simulink model "model_virtualpartner_bros"  (R2016b)
settings: Solver=FixedStepDiscrete  StartTime=0.0  StopTime=inf  FixedStep=sampleTime  RelTol=1e-3
PostLoadFcn:
  | % load model parameters
  | % pname = fileparts(get_param('model_base_bros','filename'));
  | % run([pname  '\parameters_base_model_bros.m']);
  | parameters_virtualpartner_bros;
  | 
  | % set requested state
  | set_param('model_virtualpartner_bros/Requested state','Value',num2str(0));
InitFcn:
  | % load model parameters
  | % pname = fileparts(get_param('model_base_bros','filename'));
  | % run([pname  '\parameters_base_model_bros.m']);
  | parameters_virtualpartner_bros;
  | 
  | % set requested state
  | set_param('model_virtualpartner_bros/Requested state','Value',num2str(0));
StartFcn:
  | % load model parameters
  | % pname = fileparts(get_param('model_base_bros','filename'));
  | % run([pname  '\parameters_base_model_bros.m']);
  | parameters_virtualpartner_bros;
  | 
  | % set requested state
  | set_param('model_virtualpartner_bros/Requested state','Value',num2str(0));
StopFcn:
  | % switch off data logger (to hopefully avoid corrupt files). TwinCAT doesn't properly switch off the logger when shutting down the model
  | % no idea if this'll work.
  | set_param('model_virtualpartner_bros/Record data (1 = yes, 0 = no)','Value',num2str(0));
values from neighbouring files (symbols this model uses):
  Ax = [0.0286583637244 0.0270981680387 0.0234505258969 0.0179991434705]    [data_target_signal.mat]    (also in data_target_signal3.mat = [0.0333782282668 0.0245436264839 0.0161138842629 0.007570500; data_target_signal4.mat = [0.0269405878553 0.022932388404 0.0177213023263 0.0101459636; data_target_signal5.mat = [0.0280601816416 0.0238854099083 0.0184577621273 0.010567608)
  Ay = [0.0270981680387 0.0253254894496 0.0215637914741 0.0163904070646]    [data_target_signal.mat]    (also in data_target_signal3.mat = [0.0316365733513 0.022903298684 0.0150378639378 0.0071644979; data_target_signal4.mat = [0.0262391735578 0.0220449066546 0.0169202788634 0.009702651; data_target_signal5.mat = [0.0273296180511 0.0229610462966 0.0176234498254 0.010105872)
  FFMatrix = [0 -20; 20 0]*-1    [parameters_base_model_bros.m]    (also in parameters_model_virtualpartner_bros.m = -[0 -15; 15 0]; parameters_virtualpartner_bros.m = -[0 -15; 15 0])
  Lb = 0.07    [parameters_base_model_bros.m]    (also in parameters_model_virtualpartner_bros.m; parameters_virtualpartner_bros.m)
  Lf = 0.238    [parameters_base_model_bros.m]    (also in parameters_model_virtualpartner_bros.m; parameters_virtualpartner_bros.m)
  Lu = 0.153    [parameters_base_model_bros.m]    (also in parameters_model_virtualpartner_bros.m; parameters_virtualpartner_bros.m)
  nx = [3 4 6 9]    [data_target_signal.mat]    (also in data_target_signal3.mat = [6 11 17 29]; data_target_signal4.mat = [6 11 17 29]; data_target_signal5.mat = [6 11 17 29])
  ny = [4 5 7 10]    [data_target_signal.mat]    (also in data_target_signal3.mat = [7 12 18 30]; data_target_signal4.mat = [7 12 18 30]; data_target_signal5.mat = [7 12 18 30])
  phx = [-7.77441521106 -8.5348832042 -4.36104325862 -3.78796037329]    [data_target_signal.mat]    (also in data_target_signal3.mat = [3.56575266464 -2.00335535647 1.65538939475 0.759048650391]; data_target_signal4.mat = [-7.8125213649 -4.12353525545 6.3256632478 -1.21163926456]; data_target_signal5.mat = [2.80153374524 -3.20046313064 -3.48286348128 -10.5236026319])
  phy = [-0.714244784373 -3.45250659197 3.9180169666 4.93073057512]    [data_target_signal.mat]    (also in data_target_signal3.mat = [9.98760310067 -6.16453798136 -6.84315611985 5.69872885715]; data_target_signal4.mat = [6.54917483844 9.11210927212 4.8993819932 2.56946947623]; data_target_signal5.mat = [-1.40862004251 -1.67034924642 8.20266618674 -4.37156725072])
  sampleTime = 0.001    [parameters_base_model_bros.m]    (also in parameters_model_virtualpartner_bros.m; parameters_virtualpartner_bros.m)
undefined symbols (not defined in the file or in its folder): BROS1, BROS2, VP
libraries: simulink x29, LibraryFM x14, VariousBlocksLibrary x7, simulink_extras x1
(part 3 of 3)

== system model_virtualpartner_bros/Robot2/DataToEtherCAT/WorkspacePositionGuard ==
  note: Check internal angles
  note: Check whether endpoint position is within the predefined workspace
      | (ellipse)
  note: Check for singularity of joint configuration by checking
      | the condition number. When it exceeds a certain value, go to a safe mode
      | For now, this means disabling the actuators.
      | Note that the boundaries set using admittance should prohibit this from happening.
      | However, if sometjhing really goes wrong, this is a safe guard
  BusRobot : Inport
  StateSystem : Inport  Port=2
  AvoidAlgebraicLoop : Memory
  Bus Selector : BusSelector  OutputSignals=xOpSpace.x,xOpSpace.conditioning,qJointSpace.q_all
  CheckInternalAngles : MATLAB Function  TreatAsAtomicUnit=on
  Compare To Constant : simulink/Logic and Bit Operations/Compare To Constant  relop=>  const=4  OutDataTypeStr=boolean
  Compare To Constant1 : simulink/Logic and Bit Operations/Compare To Constant  relop=>=  const=2.75  OutDataTypeStr=boolean
  Data Type Conversion1 : DataTypeConversion  OutDataTypeStr=boolean
  Data Type Conversion2 : DataTypeConversion  Commented=through  OutDataTypeStr=int32
  Data Type Conversion4 : DataTypeConversion  OutDataTypeStr=boolean
  Detect Change : simulink/Logic and Bit Operations/Detect Change  vinit=0  InputProcessing=Inherited  OutDataTypeStr=boolean
  EndpointPositionGuard : MATLAB Function  TreatAsAtomicUnit=on
  LatchRising : LibraryFM/Utilities/LatchRising  ic=0
  Logical Operator : Logic  Operator=OR  AllPortsSameDT=off  OutDataTypeStr=boolean
  Mux : Mux  Inputs=2
  ShowWorkspaceErrorLatched : Display
  WorkspaceLastError : Display
  WorkspaceError : Outport
  WorkspaceErrorLatched : Outport  Port=2
  wires:
  BusRobot/1 -> Bus Selector/1
  Bus Selector/1 -> EndpointPositionGuard/2(xe)  "<x>"
  LatchRising/1 -> Data Type Conversion2/1
  EndpointPositionGuard/1(error) -> Data Type Conversion1/1
  Mux/1 -> AvoidAlgebraicLoop/1, WorkspaceLastError/1
  Detect Change/1 -> LatchRising/Trigger
  AvoidAlgebraicLoop/1 -> WorkspaceError/1, Detect Change/1, LatchRising/1
  Compare To Constant/1 -> EndpointPositionGuard/1(correctState)
  Bus Selector/2 -> Compare To Constant1/1  "<conditioning>"
  StateSystem/1 -> Compare To Constant/1
  Data Type Conversion2/1 -> WorkspaceErrorLatched/1, ShowWorkspaceErrorLatched/1
  CheckInternalAngles/1(angleError) -> Data Type Conversion4/1
  Bus Selector/3 -> CheckInternalAngles/1(theta)  "<q_all>"
  Data Type Conversion4/1 -> Mux/2
  Logical Operator/1 -> Mux/1
  Data Type Conversion1/1 -> Logical Operator/1
  Compare To Constant1/1 -> Logical Operator/2

== system model_virtualpartner_bros/Experiment & Haptics/Admittance // Virtual model1/Virtual Model/HoldFirstSampleOnEnable ==
  note: These blocks hold the first sample of the input
      | when the block is enabled (through the action port)
  x : Inport
  Enable : EnablePort  StatesWhenEnabling=reset
  Counter Free-Running : simulink/Sources/Counter Free-Running  NumBits=32  tsamp=-1
  Display : Display
  Memory1 : Memory
  Switch : Switch  Threshold=1
  x0 : Outport
  wires:
  Switch/1 -> Display/1, Memory1/1, x0/1
  Memory1/1 -> Switch/1
  Counter Free-Running/1 -> Switch/2
  x/1 -> Switch/3

== system model_virtualpartner_bros/Experiment & Haptics/Admittance // Virtual model1/Virtual Model/HoldFirstSampleOnEnable1 ==
  note: These blocks hold the first sample of the input
      | when the block is enabled (through the action port)
  x : Inport
  Enable : EnablePort  StatesWhenEnabling=reset
  Counter Free-Running : simulink/Sources/Counter Free-Running  NumBits=32  tsamp=-1
  Display : Display
  Memory1 : Memory
  Switch : Switch  Threshold=1
  x0 : Outport
  wires:
  Switch/1 -> Display/1, Memory1/1, x0/1
  Memory1/1 -> Switch/1
  Counter Free-Running/1 -> Switch/2
  x/1 -> Switch/3

== system model_virtualpartner_bros/Experiment & Haptics/Admittance // Virtual model1/Virtual Model/simple Virtual partner LQG2 ==
  target : Inport
  L_VP : Inport  Port=2
  ExecuteVP : Inport  Port=3
  Fs : Inport  Port=4
  CoAimmstant : Constant  Value=VP.Aim
  CoAimmstant1 : Constant  Value=VP.B
  CoAimmstant2 : Constant  Value=VP.Ae
  CoAimmstant3 : Constant  Value=VP.H
  CoAimmstant5 : Constant  Value=VP.Ov
  CoAimmstant6 : Constant  Value=VP.Ow
  CoAimmstant8 : Constant  Value=VP.Ndelay
  Compare To Zero : simulink/Logic and Bit Operations/Compare To Zero  relop=>  OutDataTypeStr=boolean
  Constant : Constant  Value=VP.m
  Data Type Conversion : DataTypeConversion  OutDataTypeStr=double
  Mux : Mux  Inputs=2
  Product : Product
  Virtual Partner LQG : MATLAB Function  TreatAsAtomicUnit=on
  select [px vx py vy] from state vector : Selector  InputPortWidth=14  IndexOptions=Index vector (dialog)  Indices=[1 2 3 4]  OutputSizes=1
  xVP_prev1 : UnitDelay  InitialCondition=VP.x0  SampleTime=-1
  xhatp1 : Delay  DelayLength=1
  y1 : Delay  DelayLength=100
  x_VP : Outport
  data : Outport  Port=2
  wires:
  CoAimmstant5/1 -> Virtual Partner LQG/5(Ov)
  CoAimmstant2/1 -> Virtual Partner LQG/1(Ae)
  CoAimmstant3/1 -> Virtual Partner LQG/4(H)
  CoAimmstant1/1 -> Virtual Partner LQG/3(B)
  L_VP/1 -> Virtual Partner LQG/9(L)
  CoAimmstant/1 -> Virtual Partner LQG/2(Aim)
  xVP_prev1/1 -> Virtual Partner LQG/11(xVP_prev)
  CoAimmstant6/1 -> Virtual Partner LQG/6(Ow)
  Virtual Partner LQG/2(y) -> Mux/1, y1/1
  y1/1 -> Virtual Partner LQG/12(y_delay)
  Virtual Partner LQG/3(xhatp) -> Mux/2, xhatp1/1
  xhatp1/1 -> Virtual Partner LQG/13(xhatp_delay)
  CoAimmstant8/1 -> Virtual Partner LQG/7(Ndelay)
  target/1 -> Virtual Partner LQG/8(target)
  Virtual Partner LQG/1(x_VP) -> xVP_prev1/1, select [px vx py vy] from state vector/1
  ExecuteVP/1 -> Compare To Zero/1
  Compare To Zero/1 -> Data Type Conversion/1
  Product/1 -> x_VP/1
  select [px vx py vy] from state vector/1 -> Product/1
  Data Type Conversion/1 -> Product/2
  Mux/1 -> data/1
  Fs/1 -> Virtual Partner LQG/10(Fs)
  Constant/1 -> Virtual Partner LQG/14(m_vp)

== system model_virtualpartner_bros/Experiment & Haptics/Admittance // Virtual model1/Virtual partner control law/Triggered Subsystem ==
  VPModelParams : Inport
  Trigger : TriggerPort  VariantControl=Variant
  CoAimmstant : Constant  Value=VP.Aim
  CoAimmstant1 : Constant  Value=VP.B
  MATLAB Function : MATLAB Function  TreatAsAtomicUnit=on
  FBGains : Outport  InitialOutput=zeros(2,14)
  wires:
  VPModelParams/1 -> MATLAB Function/1(modelparams)
  MATLAB Function/1(L) -> FBGains/1
  CoAimmstant/1 -> MATLAB Function/2(Aim_vp)
  CoAimmstant1/1 -> MATLAB Function/3(B_vp)

== system model_virtualpartner_bros/Experiment & Haptics/Admittance // Virtual model1/Virtual partner control law/Triggered Subsystem1 ==
  VPModelParams : Inport
  Trigger : TriggerPort  VariantControl=Variant
  CoAimmstant : Constant  Value=VP.Aim
  CoAimmstant1 : Constant  Value=VP.B
  MATLAB Function : MATLAB Function  TreatAsAtomicUnit=on
  FBGains : Outport  InitialOutput=zeros(2,14)
  wires:
  VPModelParams/1 -> MATLAB Function/1(modelparams)
  MATLAB Function/1(L) -> FBGains/1
  CoAimmstant/1 -> MATLAB Function/2(Aim_vp)
  CoAimmstant1/1 -> MATLAB Function/3(B_vp)

== system model_virtualpartner_bros/Robot1/Controller_PD/at home/HoldFirstSampleOnEnable ==
  note: These blocks hold the first sample of the input
      | when the block is enabled (through the action port)
  x : Inport
  Enable : EnablePort  StatesWhenEnabling=reset
  Counter Free-Running : simulink/Sources/Counter Free-Running  NumBits=32  tsamp=-1
  Memory1 : Memory
  Signal Conversion : SignalConversion  OverrideOpt=off
  Switch : Switch  Threshold=1
  x0 : Outport
  wires:
  x/1 -> Switch/3
  Counter Free-Running/1 -> Switch/2
  Memory1/1 -> Switch/1
  Switch/1 -> Signal Conversion/1, Memory1/1
  Signal Conversion/1 -> x0/1

== system model_virtualpartner_bros/Robot1/DataFromEtherCAT/Calculate Arrange Joint and Op Space/forward kinematics ==
  JointPosition_rad : Inport  PortDimensions=[2 1]
  JointVelocity_rads : Inport  Port=2  PortDimensions=[2 1]
  JointAcceleration_rads2 : Inport  Port=3  PortDimensions=[2 1]
  Je : MATLAB Function  TreatAsAtomicUnit=on
  Jedot : MATLAB Function  TreatAsAtomicUnit=on
  Product : Product  Multiplication=Matrix(*)
  calculate xddot : MATLAB Function  TreatAsAtomicUnit=on
  forward kinematics : MATLAB Function  TreatAsAtomicUnit=on
  x : Outport
  xdot : Outport  Port=2
  xddot : Outport  Port=3
  J : Outport  Port=4
  Jdot : Outport  Port=5
  wires:
  JointPosition_rad/1 -> forward kinematics/1(q), Jedot/1(q), Je/1(q)
  Je/1(Je) -> calculate xddot/3(J), Product/1, J/1
  JointVelocity_rads/1 -> calculate xddot/2(qdot), Product/2, Jedot/2(qdot)
  Jedot/1(Jedot) -> calculate xddot/4(Jdot), Jdot/1
  Product/1 -> xdot/1
  forward kinematics/1(x) -> x/1
  calculate xddot/1(xddot) -> xddot/1
  JointAcceleration_rads2/1 -> calculate xddot/1(qddot)

== system model_virtualpartner_bros/Robot1/DataFromEtherCAT/Calculate Arrange Joint and Op Space/forward kinematics1 ==
  JointPosition_rad : Inport  PortDimensions=[2 1]
  JointVelocity_rads : Inport  Port=2  PortDimensions=[2 1]
  JointAcceleration_rads2 : Inport  Port=3  PortDimensions=[2 1]
  Je : MATLAB Function  TreatAsAtomicUnit=on
  Jedot : MATLAB Function  TreatAsAtomicUnit=on
  Product : Product  Multiplication=Matrix(*)
  calculate xddot : MATLAB Function  TreatAsAtomicUnit=on
  forward kinematics : MATLAB Function  TreatAsAtomicUnit=on
  x : Outport
  xdot : Outport  Port=2
  xddot : Outport  Port=3
  J : Outport  Port=4
  Jdot : Outport  Port=5
  wires:
  JointPosition_rad/1 -> forward kinematics/1(q), Jedot/1(q), Je/1(q)
  Je/1(Je) -> calculate xddot/3(J), Product/1, J/1
  JointVelocity_rads/1 -> calculate xddot/2(qdot), Product/2, Jedot/2(qdot)
  Jedot/1(Jedot) -> calculate xddot/4(Jdot), Jdot/1
  Product/1 -> xdot/1
  forward kinematics/1(x) -> x/1
  calculate xddot/1(xddot) -> xddot/1
  JointAcceleration_rads2/1 -> calculate xddot/1(qddot)

== system model_virtualpartner_bros/Robot2/Controller_PD/at home/HoldFirstSampleOnEnable ==
  note: These blocks hold the first sample of the input
      | when the block is enabled (through the action port)
  x : Inport
  Enable : EnablePort  StatesWhenEnabling=reset
  Counter Free-Running : simulink/Sources/Counter Free-Running  NumBits=32  tsamp=-1
  Memory1 : Memory
  Signal Conversion : SignalConversion  OverrideOpt=off
  Switch : Switch  Threshold=1
  x0 : Outport
  wires:
  x/1 -> Switch/3
  Counter Free-Running/1 -> Switch/2
  Memory1/1 -> Switch/1
  Switch/1 -> Signal Conversion/1, Memory1/1
  Signal Conversion/1 -> x0/1

== system model_virtualpartner_bros/Robot2/DataFromEtherCAT/Calculate Arrange Joint and Op Space/forward kinematics ==
  JointPosition_rad : Inport  PortDimensions=[2 1]
  JointVelocity_rads : Inport  Port=2  PortDimensions=[2 1]
  JointAcceleration_rads2 : Inport  Port=3  PortDimensions=[2 1]
  Je : MATLAB Function  TreatAsAtomicUnit=on
  Jedot : MATLAB Function  TreatAsAtomicUnit=on
  Product : Product  Multiplication=Matrix(*)
  calculate xddot : MATLAB Function  TreatAsAtomicUnit=on
  forward kinematics : MATLAB Function  TreatAsAtomicUnit=on
  x : Outport
  xdot : Outport  Port=2
  xddot : Outport  Port=3
  J : Outport  Port=4
  Jdot : Outport  Port=5
  wires:
  JointPosition_rad/1 -> forward kinematics/1(q), Jedot/1(q), Je/1(q)
  Je/1(Je) -> calculate xddot/3(J), Product/1, J/1
  JointVelocity_rads/1 -> calculate xddot/2(qdot), Product/2, Jedot/2(qdot)
  Jedot/1(Jedot) -> calculate xddot/4(Jdot), Jdot/1
  Product/1 -> xdot/1
  forward kinematics/1(x) -> x/1
  calculate xddot/1(xddot) -> xddot/1
  JointAcceleration_rads2/1 -> calculate xddot/1(qddot)

== system model_virtualpartner_bros/Robot2/DataFromEtherCAT/Calculate Arrange Joint and Op Space/forward kinematics1 ==
  JointPosition_rad : Inport  PortDimensions=[2 1]
  JointVelocity_rads : Inport  Port=2  PortDimensions=[2 1]
  JointAcceleration_rads2 : Inport  Port=3  PortDimensions=[2 1]
  Je : MATLAB Function  TreatAsAtomicUnit=on
  Jedot : MATLAB Function  TreatAsAtomicUnit=on
  Product : Product  Multiplication=Matrix(*)
  calculate xddot : MATLAB Function  TreatAsAtomicUnit=on
  forward kinematics : MATLAB Function  TreatAsAtomicUnit=on
  x : Outport
  xdot : Outport  Port=2
  xddot : Outport  Port=3
  J : Outport  Port=4
  Jdot : Outport  Port=5
  wires:
  JointPosition_rad/1 -> forward kinematics/1(q), Jedot/1(q), Je/1(q)
  Je/1(Je) -> calculate xddot/3(J), Product/1, J/1
  JointVelocity_rads/1 -> calculate xddot/2(qdot), Product/2, Jedot/2(qdot)
  Jedot/1(Jedot) -> calculate xddot/4(Jdot), Jdot/1
  Product/1 -> xdot/1
  forward kinematics/1(x) -> x/1
  calculate xddot/1(xddot) -> xddot/1
  JointAcceleration_rads2/1 -> calculate xddot/1(qddot)

== matlab function model_virtualpartner_bros/Robot2/Controller_PD/PD + nonlin (op space)/invJ1 ==
  data: x input; J input; y output
function y = invJ(x,J)

y = J.'*x;

== matlab function model_virtualpartner_bros/Experiment & Haptics/CalculateTrialPerformanceMSE/Calc_RMSE_BROS1 ==
  data: error input; RMSE output
function RMSE = RMSE(error)
% calculate the mean-squared error

persistent N; % number of samples, counter
persistent SSE; % sum of squared of error
if isempty(N), N = 0; end
if isempty(SSE), SSE = 0; end

N = N+1; % new datapoint, increase sample counter

SSE = SSE + norm(error)^2;
RMSE = sqrt(SSE / N);

== matlab function model_virtualpartner_bros/Robot1/DataFromEtherCAT/Calculate Arrange Joint and Op Space/Condition number ==
  data: J input; C output
function C = conditioning(J)
%#codegen

C = norm(J)*norm(pinv(J));

== matlab function model_virtualpartner_bros/Robot2/Controller_PD/PD + nonlin (op space)/nonlinear compensation ==
  data: J input; Jdot input; qdot input; tau output; RobotStruct parameter
function tau = n(J,Jdot,qdot,RobotStruct)
% mass matrix
phat = RobotStruct.DynModParams;

% select parameters
me = phat(3);
Fs1 = phat(4);
Fv1 = phat(5);
Fs2 = phat(6);
Fv2 = phat(7);

% % jacobians
% J = func_eq_Je(q(1),q(2),Lf,Lu,Lb);
% Jdot = func_eq_Jedot(q(1),q(2),qdot(1),qdot(2),Lf,Lu,Lb);

% calculate joint space mass matrix;
p = [me;Fs1;Fv1;Fs2;Fv2];

% psi 
Psi = [(J'*Jdot)*qdot [ssign(qdot(1)) qdot(1); 0 0] [0 0; ssign(qdot(2)) qdot(2)]];

% torque
tau = Psi*p;

function x = ssign(u,b)
%% x = ssign(u,b)
% soft sign
if nargin < 2
    b = 8;
end

x = 2./(1+exp(-b*u))-1;

== matlab function model_virtualpartner_bros/Robot1/DataFromEtherCAT/Calculate Arrange Joint and Op Space/forward kinematics1/Je ==
  data: q input; Je output size=[2 2]; Lf parameter; Lu parameter; Lb parameter
function Je = Je( q, Lf, Lu, Lb)
%#codegen

% Calculate the Jacobian for this particular device configuration.
% Note that the function func_eq_Je needs to be in the libraries/kinematis_functions folder

% jacobians
Je = func_eq_Je(q(1),q(2),Lf,Lu,Lb);

== matlab function model_virtualpartner_bros/Robot1/DataFromEtherCAT/Calculate Arrange Joint and Op Space/forward kinematics1/Jedot ==
  data: q input; qdot input; Jedot output size=[2 2]; Lf parameter; Lu parameter; Lb parameter
function Jedot = Jedot( q, qdot, Lf, Lu, Lb)
%#codegen

% Calculate the time derivative of the Jacobian for this particular device configuration.
% Note that the function func_eq_Je needs to be in the libraries/kinematis_functions folder


% jacobians
Jedot = func_eq_Jedot(q(1),q(2),qdot(1),qdot(2),Lf,Lu,Lb);

== matlab function model_virtualpartner_bros/Robot1/DataFromEtherCAT/Calculate Arrange Joint and Op Space/forward kinematics1/calculate xddot ==
  data: qddot input; qdot input size=[2 1]; J input; xddot output size=[2 1]; Jdot input
function xddot = calc_xddot(qddot, qdot, J, Jdot)
%#codegen

xddot = J*qddot + Jdot*qdot;

== matlab function model_virtualpartner_bros/Robot2/DataFromEtherCAT/Calculate Arrange Joint and Op Space/Condition number ==
  data: J input; C output
function C = conditioning(J)
%#codegen

C = norm(J)*norm(pinv(J));

== matlab function model_virtualpartner_bros/Experiment & Haptics/Target position ==
  data: time input; T input; time_rand input; p output; nx parameter; ny parameter; Ax parameter; Ay parameter; phx parameter; phy parameter; v output
function [p, v]  = msin_target (time, T, time_rand, nx, ny, Ax, Ay, phx, phy) 

% prepare frequencies
dw = 2*pi/T; %w0 depends on trial duration
wx = dw*nx;
wy = dw*ny;

% calculate x and y
px = 0;
py = 0;
vx = 0;
vy = 0;

% randomization
% for every multiple of 20, rotate the target signal
nRand = floor(time_rand/20);
if nRand > 5, nRand = 5; end

% add random starting time (semi-randomization)
time = time + mod(time_rand,20.0);

% calculate sum-of-sines
for i = 1:length(wx)
    % position
    px = px + Ax(i)*sin(wx(i)*time+phx(i));
    py = py + Ay(i)*sin(wy(i)*time+phy(i));
    
    % velocity
    vx = vx + Ax(i)*wx(i)*cos(wx(i)*time+phx(i));
    vy = vy + Ay(i)*wy(i)*cos(wy(i)*time+phy(i));
end

p = [px; py];
v = [vx; vy];

% due to the difference in coordiante systems (of human reaching, y
% forward, x to the right; robot: y towards you and x to the left), rotate
% the target such that it is in a human-centered coordinate system.
p = -p;
v = -v;

% rotate target (to make it more random-appearing)
thetaRot = nRand*(2*pi/6);

R = [cos(thetaRot) -sin(thetaRot); sin(thetaRot) cos(thetaRot)];

p = R*p;
v = R*v;              

end

== matlab function model_virtualpartner_bros/Robot1/DataFromEtherCAT/Calculate Arrange Joint and Op Space/forward kinematics/forward kinematics ==
  data: q input; x output size=[2 1]; Lf parameter; Lu parameter; Lb parameter
function x = FK(q, Lf, Lu, Lb)
%#codegen

% Calculate the endpoint position (forward kinematics)
% Note that the function func_eq_FK needs to be in the libraries/kinematis_functions folder


x = func_eq_FK(q(1),q(2),Lf,Lu,Lb);

== matlab function model_virtualpartner_bros/Robot1/DataFromEtherCAT/Calculate Arrange Joint and Op Space/forward kinematics1/forward kinematics ==
  data: q input; x output size=[2 1]; Lf parameter; Lu parameter; Lb parameter
function x = FK(q, Lf, Lu, Lb)
%#codegen

% Calculate the endpoint position (forward kinematics)
% Note that the function func_eq_FK needs to be in the libraries/kinematis_functions folder


x = func_eq_FK(q(1),q(2),Lf,Lu,Lb);

== matlab function model_virtualpartner_bros/Robot1/DataToEtherCAT/FTSensorError/MATLAB Function ==
  data: ForcesTorques input; e output; MaxForcesTorques input
function e = fcn(ForcesTorques, MaxForcesTorques)

% throw error when any of the forces/torques go over a max allowable value
if any(abs(ForcesTorques) > MaxForcesTorques) 
    e = 1;
else
    e = 0;
end

== matlab function model_virtualpartner_bros/Robot1/Controller_PD/PD + nonlin (op space)/invJ1 ==
  data: x input; J input; y output
function y = invJ(x,J)

y = J.'*x;

== matlab function model_virtualpartner_bros/Robot2/DataFromEtherCAT/Calculate Arrange Joint and Op Space/IK all joints ==
  data: x input; q_all output; Lf parameter; Lu parameter; Lb parameter
function q_all = IK_all(x,Lf,Lu,Lb)
%#codegen

q_all = func_eqs_IK_all(x(1),x(2),Lf,Lu,Lb);

if any(isnan(q_all)) || any(isinf(q_all))
    q_all = zeros(5,1);
end

== matlab function model_virtualpartner_bros/Robot2/DataFromEtherCAT/Calculate Arrange Joint and Op Space/forward kinematics/Je ==
  data: q input; Je output size=[2 2]; Lf parameter; Lu parameter; Lb parameter
function Je = Je( q, Lf, Lu, Lb)
%#codegen

% Calculate the Jacobian for this particular device configuration.
% Note that the function func_eq_Je needs to be in the libraries/kinematis_functions folder

% jacobians
Je = func_eq_Je(q(1),q(2),Lf,Lu,Lb);

== matlab function model_virtualpartner_bros/Robot2/DataFromEtherCAT/Calculate Arrange Joint and Op Space/forward kinematics/Jedot ==
  data: q input; qdot input; Jedot output size=[2 2]; Lf parameter; Lu parameter; Lb parameter
function Jedot = Jedot( q, qdot, Lf, Lu, Lb)
%#codegen

% Calculate the time derivative of the Jacobian for this particular device configuration.
% Note that the function func_eq_Je needs to be in the libraries/kinematis_functions folder


% jacobians
Jedot = func_eq_Jedot(q(1),q(2),qdot(1),qdot(2),Lf,Lu,Lb);

== matlab function model_virtualpartner_bros/Robot2/DataFromEtherCAT/Calculate Arrange Joint and Op Space/forward kinematics/calculate xddot ==
  data: qddot input; qdot input size=[2 1]; J input; xddot output size=[2 1]; Jdot input
function xddot = calc_xddot(qddot, qdot, J, Jdot)
%#codegen

xddot = J*qddot + Jdot*qdot;

== matlab function model_virtualpartner_bros/Robot2/DataFromEtherCAT/Calculate Arrange Joint and Op Space/forward kinematics/forward kinematics ==
  data: q input; x output size=[2 1]; Lf parameter; Lu parameter; Lb parameter
function x = FK(q, Lf, Lu, Lb)
%#codegen

% Calculate the endpoint position (forward kinematics)
% Note that the function func_eq_FK needs to be in the libraries/kinematis_functions folder


x = func_eq_FK(q(1),q(2),Lf,Lu,Lb);

== matlab function model_virtualpartner_bros/Robot1/DataFromEtherCAT/Calculate Arrange Joint and Op Space/forward kinematics/Je ==
  data: q input; Je output size=[2 2]; Lf parameter; Lu parameter; Lb parameter
function Je = Je( q, Lf, Lu, Lb)
%#codegen

% Calculate the Jacobian for this particular device configuration.
% Note that the function func_eq_Je needs to be in the libraries/kinematis_functions folder

% jacobians
Je = func_eq_Je(q(1),q(2),Lf,Lu,Lb);

== matlab function model_virtualpartner_bros/Robot1/DataFromEtherCAT/Calculate Arrange Joint and Op Space/forward kinematics/Jedot ==
  data: q input; qdot input; Jedot output size=[2 2]; Lf parameter; Lu parameter; Lb parameter
function Jedot = Jedot( q, qdot, Lf, Lu, Lb)
%#codegen

% Calculate the time derivative of the Jacobian for this particular device configuration.
% Note that the function func_eq_Je needs to be in the libraries/kinematis_functions folder


% jacobians
Jedot = func_eq_Jedot(q(1),q(2),qdot(1),qdot(2),Lf,Lu,Lb);

== matlab function model_virtualpartner_bros/Robot1/DataFromEtherCAT/FTSensor_K6D27/CorrectOffset ==
  data: u_in input; u_out output; reset input; corrected output
function [u_out,corrected] = CorrectOffset(u_in,reset)
%#codegen

persistent data_ offset_ counter_ corrected_;
N = 1000;

% initialize
if isempty(data_)
    data_ = zeros(size(u_in,1), N);
    offset_ = zeros(size(u_in));
    counter_ = 1;
    corrected_ = 0;
end

if (counter_ <= N)
    data_(:,counter_) = u_in;
end

counter_ = counter_ + 1;
if reset
    counter_ = 1;
end

% calculate mean
if counter_ == N
    corrected_ = 1;
    offset_ = mean(data_,2);
end

corrected = corrected_;
u_out = u_in - offset_;

== matlab function model_virtualpartner_bros/Robot2/DataFromEtherCAT/Calculate Arrange Joint and Op Space/forward kinematics1/Je ==
  data: q input; Je output size=[2 2]; Lf parameter; Lu parameter; Lb parameter
function Je = Je( q, Lf, Lu, Lb)
%#codegen

% Calculate the Jacobian for this particular device configuration.
% Note that the function func_eq_Je needs to be in the libraries/kinematis_functions folder

% jacobians
Je = func_eq_Je(q(1),q(2),Lf,Lu,Lb);

== matlab function model_virtualpartner_bros/Robot1/DataFromEtherCAT/Calculate Arrange Joint and Op Space/IK all joints ==
  data: x input; q_all output; Lf parameter; Lu parameter; Lb parameter
function q_all = IK_all(x,Lf,Lu,Lb)
%#codegen

q_all = func_eqs_IK_all(x(1),x(2),Lf,Lu,Lb);

if any(isnan(q_all)) || any(isinf(q_all))
    q_all = zeros(5,1);
end

== matlab function model_virtualpartner_bros/Robot1/DataFromEtherCAT/Calculate Arrange Joint and Op Space/forward kinematics/calculate xddot ==
  data: qddot input; qdot input size=[2 1]; J input; xddot output size=[2 1]; Jdot input
function xddot = calc_xddot(qddot, qdot, J, Jdot)
%#codegen

xddot = J*qddot + Jdot*qdot;

== matlab function model_virtualpartner_bros/Robot2/DataFromEtherCAT/Calculate Arrange Joint and Op Space/forward kinematics1/Jedot ==
  data: q input; qdot input; Jedot output size=[2 2]; Lf parameter; Lu parameter; Lb parameter
function Jedot = Jedot( q, qdot, Lf, Lu, Lb)
%#codegen

% Calculate the time derivative of the Jacobian for this particular device configuration.
% Note that the function func_eq_Je needs to be in the libraries/kinematis_functions folder


% jacobians
Jedot = func_eq_Jedot(q(1),q(2),qdot(1),qdot(2),Lf,Lu,Lb);

== matlab function model_virtualpartner_bros/Robot1/Controller_PD/PD + nonlin (op space)/nonlinear compensation ==
  data: J input; Jdot input; qdot input; tau output; RobotStruct parameter
function tau = n(J,Jdot,qdot,RobotStruct)
% mass matrix
phat = RobotStruct.DynModParams;

% select parameters
me = phat(3);
Fs1 = phat(4);
Fv1 = phat(5);
Fs2 = phat(6);
Fv2 = phat(7);

% % jacobians
% J = func_eq_Je(q(1),q(2),Lf,Lu,Lb);
% Jdot = func_eq_Jedot(q(1),q(2),qdot(1),qdot(2),Lf,Lu,Lb);

% calculate joint space mass matrix;
p = [me;Fs1;Fv1;Fs2;Fv2];

% psi 
Psi = [(J'*Jdot)*qdot [ssign(qdot(1)) qdot(1); 0 0] [0 0; ssign(qdot(2)) qdot(2)]];

% torque
tau = Psi*p;

function x = ssign(u,b)
%% x = ssign(u,b)
% soft sign
if nargin < 2
    b = 8;
end

x = 2./(1+exp(-b*u))-1;

== matlab function model_virtualpartner_bros/Robot2/DataFromEtherCAT/Calculate Arrange Joint and Op Space/forward kinematics1/calculate xddot ==
  data: qddot input; qdot input size=[2 1]; J input; xddot output size=[2 1]; Jdot input
function xddot = calc_xddot(qddot, qdot, J, Jdot)
%#codegen

xddot = J*qddot + Jdot*qdot;

== matlab function model_virtualpartner_bros/Robot2/DataFromEtherCAT/Calculate Arrange Joint and Op Space/forward kinematics1/forward kinematics ==
  data: q input; x output size=[2 1]; Lf parameter; Lu parameter; Lb parameter
function x = FK(q, Lf, Lu, Lb)
%#codegen

% Calculate the endpoint position (forward kinematics)
% Note that the function func_eq_FK needs to be in the libraries/kinematis_functions folder


x = func_eq_FK(q(1),q(2),Lf,Lu,Lb);

== matlab function model_virtualpartner_bros/Robot2/DataFromEtherCAT/FTSensor_K6D27/CorrectOffset ==
  data: u_in input; u_out output; reset input; corrected output
function [u_out,corrected] = CorrectOffset(u_in,reset)
%#codegen

persistent data_ offset_ counter_ corrected_;
N = 1000;

% initialize
if isempty(data_)
    data_ = zeros(size(u_in,1), N);
    offset_ = zeros(size(u_in));
    counter_ = 1;
    corrected_ = 0;
end

if (counter_ <= N)
    data_(:,counter_) = u_in;
end

counter_ = counter_ + 1;
if reset
    counter_ = 1;
end

% calculate mean
if counter_ == N
    corrected_ = 1;
    offset_ = mean(data_,2);
end

corrected = corrected_;
u_out = u_in - offset_;

== matlab function model_virtualpartner_bros/Robot2/DataFromEtherCAT/FTSensor_K6D27/SensorToOperationalSpace ==
  data: q_all input; Fs input; FTOpSpace output; transmatside input
function FTOpSpace = ForceSensorToOperationalSpace(q_all,Fs,transmatside)
%#codegen
q1 = q_all(1);
q2 = q_all(2);
q4 = q_all(4);
q5 = q_all(5);

% based on which arm the force sensor is connected
switch transmatside
    case 1
        alpha = pi-q2;   
        beta = q1+alpha-pi/2;
        R0 = rotmat(beta);
        R = blkdiag(R0,R0); % transform forces and moments
    case 2
        alpha = -(pi - q4);
        beta = q5+alpha-pi/2;
        R0 = rotmat(beta);
        R = blkdiag(R0,R0); % transform forces and moments
    otherwise
        R = eye(length(Fs));
end

% transform force
FTOpSpace = R*Fs;

function R = rotmat(q)

R = [cos(q) -sin(q) 0;...
      sin(q)  cos(q) 0;...
      0       0      1];

== matlab function model_virtualpartner_bros/Robot2/DataToEtherCAT/CreateSingleErrorValue1/ErrorToPower2 ==
  data: u input; e output
function e = errorToPowerOf2(u)

e = (2.^(0:length(u)-1))*u;

== matlab function model_virtualpartner_bros/Robot2/DataToEtherCAT/CreateSingleErrorValue2/ErrorToPower2 ==
  data: u input; e output
function e = errorToPowerOf2(u)

e = (2.^(0:length(u)-1))*u;

== matlab function model_virtualpartner_bros/Robot2/DataToEtherCAT/FTSensorError/MATLAB Function ==
  data: ForcesTorques input; e output; MaxForcesTorques input
function e = fcn(ForcesTorques, MaxForcesTorques)

% throw error when any of the forces/torques go over a max allowable value
if any(abs(ForcesTorques) > MaxForcesTorques) 
    e = 1;
else
    e = 0;
end

== matlab function model_virtualpartner_bros/Robot2/DataToEtherCAT/WorkspacePositionGuard/CheckInternalAngles ==
  data: theta input; angleError output
function angleError = checkInternalErrors(theta)
%#codegen


angleError = 0;
if any(theta([2 4]) >= 0.95*pi)
    angleError = 1;
end

== matlab function model_virtualpartner_bros/Robot2/DataToEtherCAT/WorkspacePositionGuard/EndpointPositionGuard ==
  data: correctState input; xe input; error output
function error = fcn(correctState, xe)
%#codegen


error = 0;

% only check workspace boundaries after homing state is done
if ~correctState 
    return; 
end

% x0 = 0;
% y0 = 0.2354;
% a = 0.11;
% b = 0.08;

% workspace (see design document)
x0 = 0;
y0 = 0.25024;
a = 0.1746;
b = 0.13;%0.1048;

% check if endpoint is outside a predefined ellipse
x = xe(1);
y = xe(2);

% workspace is defined as an ellipse
e = (x-x0)^2 / a^2 + (y-y0)^2 / b^2;

% if is larger than 1, the endpoint is outside the workspace
if e > 1
    error = 1;
end

== matlab function model_virtualpartner_bros/Experiment & Haptics/Admittance // Virtual model1/Virtual partner control law/Triggered Subsystem/MATLAB Function ==
  data: modelparams input; L output; Aim_vp input; B_vp input
function L = getControlLaw(modelparams, Aim_vp, B_vp)

% model parameters
wp = modelparams(1);
wv = modelparams(2);
wf = modelparams(3);
r = 1e-8;

Q = zeros(size(Aim_vp));
R = zeros(size(B_vp,2),size(B_vp,2));

% terminal cost & running cost
Q(1:14,1:14) = diag([0 0 wv wv wf wf 0 0 0 0 wp wp wp wp]);
Q(13,11) = -wp;
Q(14,12) = -wp;
Q(11,13) = -wp;
Q(12,14) = -wp;

R(1,1,:) = r;
R(2,2,:) = r;

N = 23000;

% controllaw_vp_infinitehorizon
L = controllaw_vp_infinitehorizon(Aim_vp,B_vp,Q,R,N);

== matlab function model_virtualpartner_bros/Experiment & Haptics/Admittance // Virtual model1/Virtual partner control law/Triggered Subsystem1/MATLAB Function ==
  data: modelparams input; L output; Aim_vp input; B_vp input
function L = getControlLaw(modelparams, Aim_vp, B_vp)

% model parameters
wp = modelparams(1);
wv = modelparams(2);
wf = modelparams(3);
r = 1e-8;

Q = zeros(size(Aim_vp));
R = zeros(size(B_vp,2),size(B_vp,2));

% terminal cost & running cost
Q(1:14,1:14) = diag([0 0 wv wv wf wf 0 0 0 0 wp wp wp wp]);
Q(13,11) = -wp;
Q(14,12) = -wp;
Q(11,13) = -wp;
Q(12,14) = -wp;

R(1,1,:) = r;
R(2,2,:) = r;

N = 23000;

% controllaw_vp_infinitehorizon
L = controllaw_vp_infinitehorizon(Aim_vp,B_vp,Q,R,N);

== matlab function model_virtualpartner_bros/Experiment & Haptics/CalculateTrialPerformanceMSE/Calc_RMSE_BROS2 ==
  data: error input; RMSE output
function RMSE = RMSE(error)
% calculate the mean-squared error

persistent N; % number of samples, counter
persistent SSE; % sum of squared of error
if isempty(N), N = 0; end
if isempty(SSE), SSE = 0; end

N = N+1; % new datapoint, increase sample counter

SSE = SSE + norm(error)^2;
RMSE = sqrt(SSE / N);

== matlab function model_virtualpartner_bros/Robot1/DataToEtherCAT/CreateSingleErrorValue2/ErrorToPower2 ==
  data: u input; e output
function e = errorToPowerOf2(u)

e = (2.^(0:length(u)-1))*u;

== matlab function model_virtualpartner_bros/Robot1/DataToEtherCAT/CreateSingleErrorValue1/ErrorToPower2 ==
  data: u input; e output
function e = errorToPowerOf2(u)

e = (2.^(0:length(u)-1))*u;

== matlab function model_virtualpartner_bros/Experiment & Haptics/Admittance // Virtual model1/Virtual Model/simple Virtual partner LQG2/Virtual Partner LQG ==
  data: Ae input; Aim input; B input; H input; Ov input; Ow input; Ndelay input; target input; L input; Fs input; x_VP output; y output; xVP_prev input; y_delay input size=[size(VP.H,1),1]; xhatp_delay input size=[size(VP.Ae,1), 1]; xhatp output; m_vp input
function [x_VP,y,xhatp] = fcn(Ae,Aim,B,H,Ov,Ow,Ndelay,target,L,Fs,xVP_prev,y_delay,xhatp_delay,m_vp)
noise = 0;

% persistent variables
persistent P u;
if isempty(P), P = zeros(size(Ae)); end
if isempty(u), u = zeros(2,100); end;

nX = size(Ae,1);
nY = size(H,1);

% LQG %

% calculate kalman gain
K = (P*H.')/(H*P*H.'+Ov);

% update the state uncertainty
P = (eye(nX)-K*H)*P;
% estimate new state uncertainty (for next time step)
P = Aim*P*Aim.' + Ow;

% posterior state estimate
xhat = xhatp_delay + K*(y_delay-H*xhatp_delay);

% forward projection to compensate for delay
x_comp = xhat;
for s = 1:Ndelay
    x_comp = Ae*x_comp+B*u(:,end+1-s);
end

% simulate internal model: priori state estimate
xhatp = Aim*xhat + B*u(:,end);

% control input
uk = -L*x_comp;
u = [uk u(:,1:end-1)]; % add u to input buffer, throw out old u value

% simulate real system
x_VP = Ae*xVP_prev + B*uk + [0;0;-Fs(1)*0.001/m_vp(1,1);-Fs(2)*0.001/m_vp(2,2);0;0;0;0;0;0;0;0;0;0]; 

% set target
x_VP(7:10) = target;

% observation (not delayed, this is done in the delay block outside of this
% function)
y = H*x_VP + noise*sqrt(Ov)*randn(nY,1); 

end

== matlab function model_virtualpartner_bros/Robot1/DataFromEtherCAT/FTSensor_K6D27/SensorToOperationalSpace ==
  data: q_all input; Fs input; FTOpSpace output; transmatside input
function FTOpSpace = ForceSensorToOperationalSpace(q_all,Fs,transmatside)
%#codegen
q1 = q_all(1);
q2 = q_all(2);
q4 = q_all(4);
q5 = q_all(5);

% based on which arm the force sensor is connected
switch transmatside
    case 1
        alpha = pi-q2;   
        beta = q1+alpha-pi/2;
        R0 = rotmat(beta);
        R = blkdiag(R0,R0); % transform forces and moments
    case 2
        alpha = -(pi - q4);
        beta = q5+alpha-pi/2;
        R0 = rotmat(beta);
        R = blkdiag(R0,R0); % transform forces and moments
    otherwise
        R = eye(length(Fs));
end

% transform force
FTOpSpace = R*Fs;

function R = rotmat(q)

R = [cos(q) -sin(q) 0;...
      sin(q)  cos(q) 0;...
      0       0      1];

== matlab function model_virtualpartner_bros/Experiment & Haptics/Admittance // Virtual model1/Virtual Model/Virtual model ==
  data: divTs input; x1 output; xdot1 output; xddot1 output; x2 output size=[2 1]; xdot2 output; xddot2 output; M_v input; B_v input; F1 input; F2 input; x0_1 input; x0_2 input; x1_nompos input; x2_nompos input; Kp_s input; Kd_s input; isConnected input; FFMatrix input; doForceField input; x_VP1 input; x_VP2 input; ExecuteVP_BROS1 input; ExecuteVP_BROS2 input; x1_prev input size=2; xdot1_prev input size=2; x2_prev input; xdot2_prev input; sampleTime parameter; Fs1 output; Fs2 output
function [x1,xdot1,xddot1,x2,xdot2,xddot2,Fs1,Fs2] = AC(divTs,M_v,B_v,F1,F2,...                         % time div, virtual mass, virtual damping, force sensor 1 & 2
                                                            x0_1,x0_2,x1_nompos,x2_nompos,...
                                                            Kp_s,Kd_s,isConnected,...
                                                            FFMatrix,doForceField,...
                                                            x_VP1,x_VP2,...
                                                            ExecuteVP_BROS1,ExecuteVP_BROS2,...
                                                            x1_prev,xdot1_prev,x2_prev,xdot2_prev,...
                                                            sampleTime)
                                                        
% constants & limits
div_Ts = max(1,divTs);
Ts = sampleTime/div_Ts;
maxRadius = 0.1;
maxVel = 2.0;
maxAcc = 100.0;
maxForceSpring = 50;
b_b = 0.5; % damping on workspace boundary

% persistents
persistent x1_prev_tmp x2_prev_tmp;
persistent onBoundary1 onBoundary2;

if isempty(x1_prev_tmp), x1_prev_tmp = x0_1;
else, x1_prev_tmp = x1_prev; end 
if isempty(x2_prev_tmp), x2_prev_tmp = x0_2;
else, x2_prev_tmp = x2_prev; end 

if isempty(onBoundary1), onBoundary1 = 0; end
if isempty(onBoundary2), onBoundary2 = 0; end

% lower bounds to mass and damping
m_v = max(0.05,M_v); %lower bound M_v
b_v = max(0,B_v);

if length(m_v) == 1
    m_v1 = m_v;
    m_v2 = m_v;
else
    m_v1 = m_v(1);
    m_v2 = m_v(2);
end

if length(b_v) == 1
    b_v1 = b_v;
    b_v2 = b_v;
else
    b_v1 = b_v(1);
    b_v2 = b_v(2);
end

% assign previous values to x1, x2, xdot1 etc
x1 = x1_prev;
x2 = x2_prev;
xdot1 = xdot1_prev;
xdot2 = xdot1_prev;
xddot1 = [0;0];
xddot2 = [0;0];
Fs1 = [0;0];
Fs2 = [0;0];

% perform integration of virtual dynamics
% using semi-implicit Euler integration
for ii = 1:div_Ts
    % force -> acc %

    % spring force
    if ExecuteVP_BROS1
%         Fs1 = Kp_s*(x_VP1(1:2) - x1_prev) + Kd_s*(x_VP1(3:4) - xdot1_prev);
        Fs1 = Kp_s*(x_VP1(1:2)-[0;-0.25] - x1_prev) + Kd_s*(x_VP1(3:4) - xdot1_prev);
        Fs1 = limit(Fs1,maxForceSpring);
    else
        Fs1 = [0;0];
    end
    if ExecuteVP_BROS2
        Fs2 = Kp_s*(x_VP2(1:2) - x2_prev) + Kd_s*(x_VP2(3:4) - xdot2_prev);
        Fs2 = limit(Fs2,maxForceSpring);
    else
        Fs2 = [0;0];
    end
    
    % BROS 1
    xddot1 = (F1 + isConnected*Fs1 + doForceField*FFMatrix*xdot1_prev - b_v1*xdot1_prev - onBoundary1*b_b*xdot1_prev)/m_v1;
    xddot1 = limit(xddot1,maxAcc);
    % BROS 2
    xddot2 = (F2 + isConnected*Fs2 + doForceField*FFMatrix*xdot2_prev - b_v2*xdot2_prev - onBoundary2*b_b*xdot2_prev)/m_v2;
    xddot2 = limit(xddot2,maxAcc);

    % acc -> vel %
    [xdot1, xddot1] = acc2vel(xdot1_prev,xddot1,Ts,maxVel); % BROS 1
    [xdot2, xddot2] = acc2vel(xdot2_prev,xddot2,Ts,maxVel); % BROS 2

    % vel -> pos %
    [x1,xdot1,xddot1,onBoundary1] = vel2pos(x1_prev_tmp,xdot1,xddot1,Ts,x1_nompos,maxRadius); % BROS 1
    [x2,xdot2,xddot2,onBoundary2] = vel2pos(x2_prev_tmp,xdot2,xddot2,Ts,x2_nompos,maxRadius); % BROS 1
    
    x1_prev_tmp = x1;
    x2_prev_tmp = x2;
    xdot1_prev = xdot1;
    xdot2_prev = xdot2;
end

end

function [y,lim] = limit(x,maxVal)
%% function [y,lim] = limit(x,maxVal)
    vecLen = norm(x);
    if vecLen > maxVal
        y = x / vecLen * maxVal;
        lim = 1; 
    else
        y = x;
        lim = 0;
    end
end

function [xdot, xddot] = acc2vel(xdot_prev,xddot,Ts,maxVel)
%% function [xdot, xddot] = integrate(xdot_prev,xddot,maxVel)

xdot = xdot_prev + xddot*Ts;
[xdot,lim_vel] = limit(xdot,maxVel);

if (lim_vel)
    xddot = [0;0];
end

end

function [x,xdot,xddot,onBoundary] = vel2pos(x_prev,xdot,xddot,Ts,x_nompos,maxRadius)
%% function [xdot, xddot] = integrate(xdot_prev,xddot,maxVel)
x = x_prev + xdot*Ts;

[x,lim_pos] = limit(x-x_nompos,maxRadius);
if (lim_pos)
    onBoundary = 1;
    unitVec = x/norm(x);
    xdot = xdot - dot(unitVec,xdot)*unitVec;     % remove normal component
    xddot = xddot - dot(unitVec,xddot)*unitVec;  % remove normal component 
else
    onBoundary = 0;
end
x = x + x_nompos;

end

== matlab function model_virtualpartner_bros/Robot1/DataToEtherCAT/WorkspacePositionGuard/CheckInternalAngles ==
  data: theta input; angleError output
function angleError = checkInternalErrors(theta)
%#codegen


angleError = 0;
if any(theta([2 4]) >= 0.95*pi)
    angleError = 1;
end

== matlab function model_virtualpartner_bros/Robot1/DataToEtherCAT/WorkspacePositionGuard/EndpointPositionGuard ==
  data: correctState input; xe input; error output
function error = fcn(correctState, xe)
%#codegen


error = 0;

% only check workspace boundaries after homing state is done
if ~correctState 
    return; 
end

% x0 = 0;
% y0 = 0.2354;
% a = 0.11;
% b = 0.08;

% workspace (see design document)
x0 = 0;
y0 = 0.25024;
a = 0.1746;
b = 0.13;%0.1048;

% check if endpoint is outside a predefined ellipse
x = xe(1);
y = xe(2);

% workspace is defined as an ellipse
e = (x-x0)^2 / a^2 + (y-y0)^2 / b^2;

% if is larger than 1, the endpoint is outside the workspace
if e > 1
    error = 1;
end
